simulink model "SMC_Observadores_chattering"  (R2026b)
settings: Solver=ode4  StopTime=20  FixedStep=0.0001
settings Model: Creator=nestorhernandezcastellanos  LastModifiedBy=nestorhernandezcastellanos

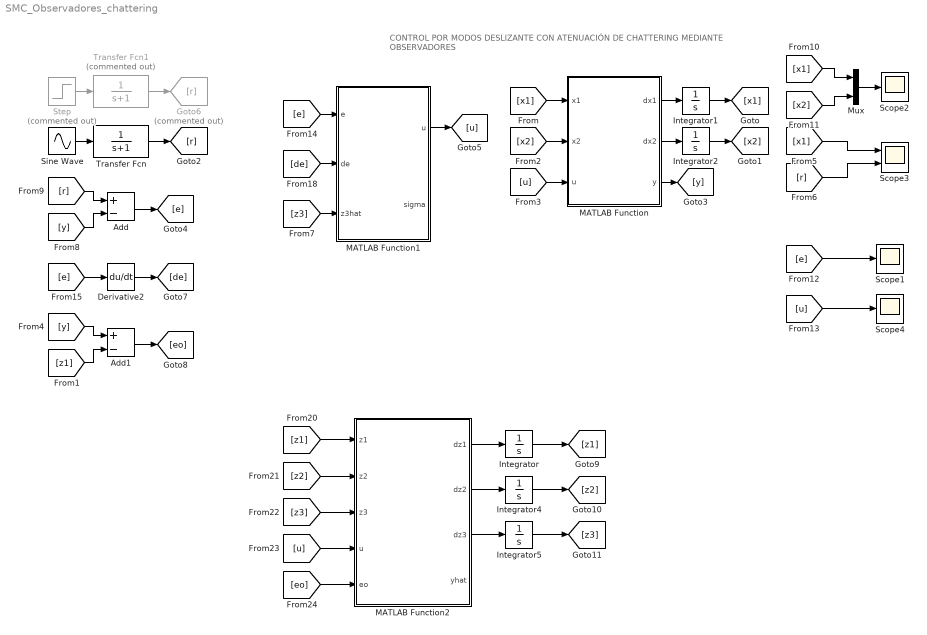
== system SMC_Observadores_chattering ==
  note: CONTROL POR MODOS DESLIZANTE CON ATENUACIÓN DE CHATTERING MEDIANTE OBSERVADORES
  Add : Sum  Inputs=+-
  Add1 : Sum  Inputs=+-
  Derivative2 : Derivative
  Goto6 : Goto  Commented=on  GotoTag=r
  Integrator : Integrator
  Integrator1 : Integrator  InitialCondition=1
  Integrator2 : Integrator  InitialCondition=-2
  Integrator4 : Integrator
  Integrator5 : Integrator
  MATLAB Function : MATLAB Function  TreatAsAtomicUnit=on
  MATLAB Function1 : MATLAB Function  TreatAsAtomicUnit=on
  MATLAB Function2 : MATLAB Function  TreatAsAtomicUnit=on
  Mux : Mux  Inputs=2
  Scope1 : Scope
      settings: ActiveDisplayYMinimum=-1.1345018827917306  ActiveDisplayYMaximum=0.21051694512557476
  Scope2 : Scope
      settings: ActiveDisplayYMinimum=-2.3780113002128531  ActiveDisplayYMaximum=1.4021017019156774  DataLoggingVariableName=ScopeData2
  Scope3 : Scope  NumInputPorts=2
      settings: ActiveDisplayYMinimum=-1.2500450787630573  ActiveDisplayYMaximum=1.2500253036424773  DataLoggingVariableName=ScopeData3
  Scope4 : Scope
      settings: ActiveDisplayYMinimum=-26.249333606618752  ActiveDisplayYMaximum=26.244002459568783
  Sine Wave : Sin  SampleTime=0
  Step : Step  Commented=on  Time=10  SampleTime=0
  Transfer Fcn : TransferFcn  Denominator=[1 1]
  Transfer Fcn1 : TransferFcn  Commented=on  Denominator=[1 1]
  wires:
  MATLAB Function/2(dx2) -> Integrator2/1
  MATLAB Function/1(dx1) -> Integrator1/1
  Mux/1 -> Scope2/1
  [de] -> MATLAB Function1/2(de)
  [x1] -> MATLAB Function/1(x1)
  [x2] -> MATLAB Function/2(x2)
  [x1] -> Scope3/1
  [r] -> Scope3/2
  Integrator2/1 -> [x2]
  Integrator1/1 -> [x1]
  MATLAB Function/3(y) -> [y]
  [y] -> Add/2
  [r] -> Add/1
  [x2] -> Mux/2
  [x1] -> Mux/1
  [e] -> Scope1/1
  [u] -> Scope4/1
  Add/1 -> [e]
  [e] -> MATLAB Function1/1(e)
  Step/1 -> Transfer Fcn1/1
  [e] -> Derivative2/1
  Derivative2/1 -> [de]
  MATLAB Function2/1(dz1) -> Integrator/1
  MATLAB Function2/2(dz2) -> Integrator4/1
  MATLAB Function2/3(dz3) -> Integrator5/1
  Integrator/1 -> [z1]
  Integrator4/1 -> [z2]
  Integrator5/1 -> [z3]
  [z1] -> MATLAB Function2/1(z1)
  [z2] -> MATLAB Function2/2(z2)
  [z3] -> MATLAB Function2/3(z3)
  [u] -> MATLAB Function2/4(u)
  [eo] -> MATLAB Function2/5(eo)
  Sine Wave/1 -> Transfer Fcn/1
  Transfer Fcn/1 -> [r]
  MATLAB Function1/1(u) -> [u]
  [u] -> MATLAB Function/3(u)
  Transfer Fcn1/1 -> Goto6/1
  Add1/1 -> [eo]
  [y] -> Add1/1
  [z1] -> Add1/2
  [z3] -> MATLAB Function1/3(z3hat)

== matlab function SMC_Observadores_chattering/MATLAB Function1 ==
  data: e input; de input; z3hat input; u output; sigma output
function [u, sigma] = controlador(e, de, z3hat)

m = ;
K = ;

% Superficie de deslizamiento
sigma = de + m*e;

% Ley de control
u = -z3hat + m*de + K*sign(sigma);

== matlab function SMC_Observadores_chattering/MATLAB Function ==
  data: x1 input; x2 input; dx1 output; u input; dx2 output; y output
function [dx1, dx2, y] = planta(x1, x2, u)

dx1 = x2;
dx2 = sin(x1*x2) + cos(x1+x2) + u;

y = x1;

== matlab function SMC_Observadores_chattering/MATLAB Function2 ==
  data: z1 input; z2 input; z3 input; u input; dz1 output; eo input; dz2 output; dz3 output; yhat output
function [dz1, dz2, dz3, yhat] = LESO(z1, z2, z3, u, eo)

Ko1 = ;
Ko2 = ;
Ko3 = ;

% Observador
dz1 = z2 + Ko1*eo;
dz2 = z3 + u + Ko2*eo;
dz3 = Ko3*eo;

% Salida estimada
yhat = z1;
